simulink subsystem "vehicleSpeed"  (R2023b)
settings: Solver=VariableStepAuto  StartTime=0.0  StopTime=10.0  RelTol=1e-3
libraries: Raptor_lib x1, wheelSpeed_lib x1
settings Model: Creator=serga  LastModifiedBy=serga

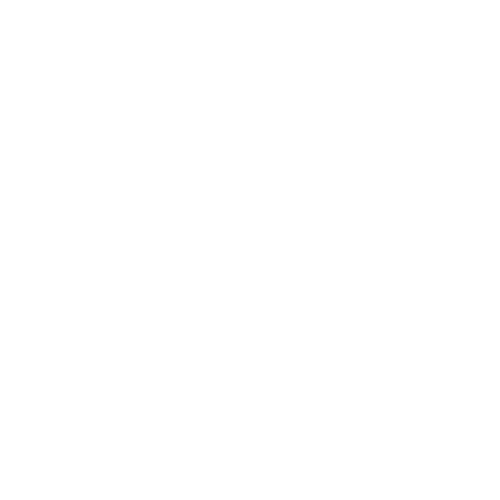
[thumbnail: Simulink's stored preview of the top-level diagram]
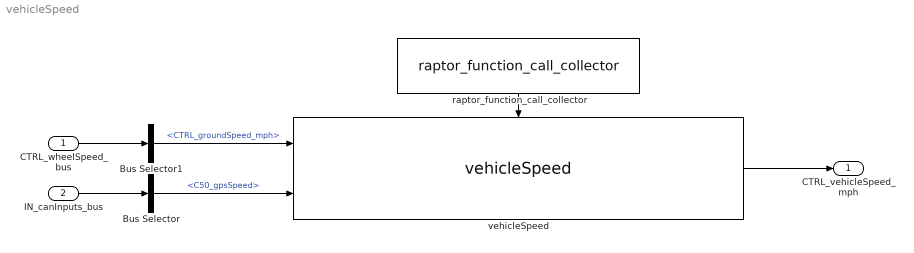
== system vehicleSpeed ==
  CTRL_wheelSpeed_bus : Inport
  IN_canInputs_bus : Inport  Port=2
  Bus Selector : BusSelector  OutputSignals=IN_can1Inputs_bus.CAN1_c50_bus.CAN1_c50_451_bus.C50_gpsSpeed
  Bus Selector1 : BusSelector  OutputSignals=CTRL_groundSpeed_mph
  raptor_function_call_collector : Raptor_lib/Triggers/raptor_function_call_collector  count=5
      settings: SourceProductName=Raptor
  vehicleSpeed : wheelSpeed_lib/vehicleSpeed  SystemSampleTime=-1  VariantActivationTime=update diagram  AllowFlexibleInterface=on  Latency=0  AutoFrameSizeCalculation=off
  CTRL_vehicleSpeed_mph : Outport
  wires:
  IN_canInputs_bus/1 -> Bus Selector/1
  CTRL_wheelSpeed_bus/1 -> Bus Selector1/1
  Bus Selector/1 -> vehicleSpeed/2  "<C50_gpsSpeed>"
  Bus Selector1/1 -> vehicleSpeed/1  "<CTRL_groundSpeed_mph>"
  raptor_function_call_collector/1 -> vehicleSpeed/Trigger
  vehicleSpeed/1 -> CTRL_vehicleSpeed_mph/1
